simulink model "Noh_Nofusion"  (R2020b)
settings: Solver=FixedStepAuto  StartTime=0.0  StopTime=Inf  FixedStep=0.01  RelTol=1e-3
PostLoadFcn:
  | if any(exist('dsrtsu_mdlpostloadfcn', 'file') ~= 0), dsrtsu_mdlpostloadfcn('Execute', bdroot); end
InitFcn:
  | , if any(exist('rtifpga_mdlclblib', 'file') ~= 0), rtifpga_mdlclblib('Init', bdroot); end,
  | , if any(exist('dsmpb_private', 'file') ~= 0), dsmpb_private('dsmpb_mdlclblib', 'Init', bdroot); end,
undefined symbols (not defined in the file): ACC_TimeGap_DecSetSwt, ACC_TimeGap_IncSetSwt, AccelPedalPosn, AccelPedalPosnVldty, AccelPedlPosnDiagc, AccPedalOverride, ACU_ShiftInProgress, ADAS_Posn_CurLane, AESSwtReq, ALC_SwtReq, BrkPedalSts, CC_ACC_CANCEL_OFFSwt, CC_ACC_CRUISE_OFFSwt, CC_ACC_DecSetSpd_SetSwt, CC_ACC_IncSetSpd_ResuSwt, CC_ACCSwtErr, CharSpd_ms, CSA_NODE, CURRENT_GEAR, CurrentGearValid, DiscIntNeverNeededParam, DrvDoorSts, DrvSBR, DrvTrqReqOvld, ECMACCInterface, ECMRespACC, ELKSwtReq, EngLimpHomeSts, EngSpd, EngState, EngState_PHEV, EngTrqMaxActSpd, EngTrqMinAct, EPS_DrvInpTrqVal_HighReslolution, EPS_FailSts, EPS_LKATorqOvrlDlvd, EPS_LKATorqOvrlDlvdVld, EPS_LKATrqOvlDlvdSts, EPS_SteerMod, EPS_TrqSnsrSts, EQ4_APPINFO, EQ4_LA_ELEM, EQ4_LA_HDR, EQ4_LAP_ELEM, EQ4_LAP_HDR, EQ4_LH_ELEM, EQ4_LH_HDR, EQ4_LRE_ELEM, EQ4_LRE_HDR, ESS_PedSwtReq, ESS_VehSwtReq, FFogLmpSts_F_Pbox, FLWheelDriveDirection, FLWheelSpd, FrntWiprSwtSts, FrntWshrSwtSts, FRWheelDriveDirection, FRWheelSpd, HazardLmpSwtSts, HCU_AccelPedalPosn_Diag ... (+153)
libraries: simulink x132, dsmpblib x27
(part 4 of 14)

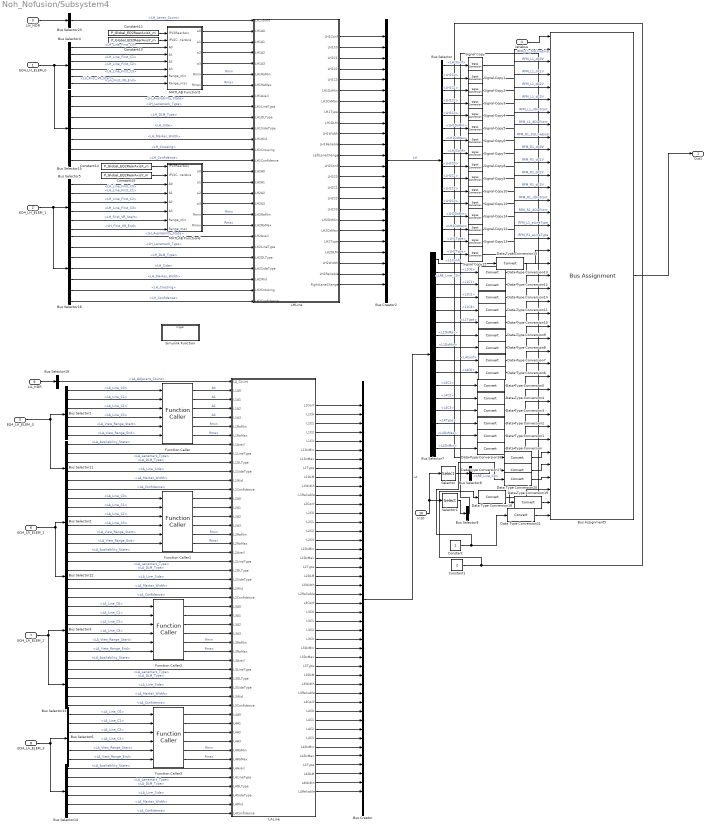
== system Noh_Nofusion/Subsystem4 ==
  EQ4_LH_ELEM_0 : Inport
  EQ4_LH_ELEM_1 : Inport  Port=2
  LH_HDR : Inport  Port=3
  lanebus : Inport  Port=4
  EQ4_LA_ELEM_0 : Inport  Port=5
  EQ4_LA_ELEM_1 : Inport  Port=6
  EQ4_LA_ELEM_2 : Inport  Port=7
  EQ4_LA_ELEM_3 : Inport  Port=8
  LA_HDR : Inport  Port=9
  In10 : Inport  Port=10
  Bus Assignment5 : BusAssignment  AssignedSignals=RFM_LINE_L1.bIsLineExist,RFM_LINE_L1.dC0V,RFM_LINE_L1.dC1V,RFM_LINE_L1.dC2V,RFM_LINE_L1.dC3V,RFM_LINE_L1.dDisStart,RFM_LINE_L1.dDisFront,RFM_LINE_R1.bIsLineExist,RFM_LINE_R1.dC0V,RFM_LINE_R1.dC1V,RFM_LINE_R1.dC2V,RFM_LINE_R1.dC3V,RFM_LINE_R1.dDisStart,RFM_LINE_R1.dDisFront,RFM_LINE_L1.eLineType,RFM_LINE_R1.eLineType,RFM_LINE_L2.bIsLineExist,RFM_LINE_L2.dC0V,RFM_LINE_L2.dC1V,RFM_LINE_L2.dC2V,RFM_LINE_L2.dC3V,RFM_LINE_L2.eLineType,RFM_LINE_L2.dDisFront,RFM_LINE_L2.dDisStart,RFM_LINE_R2.bIsLineExist,RFM_LINE_R2.dC0V,RFM_LINE_R2.dC1V,RFM_LINE_R2.dC2V,RFM_LINE_R2.dC3V,RFM_LINE_R2.eLineType,RFM_LINE_R2.dDisStart,RFM_LINE_R2.dDisFront,RFM_LINE_LB.bIsLineExist,RFM_LINE_LB.dC0V,RFM_LINE_LB.eLineType,RFM_LINE_RB.bIsLineExist,RFM_LINE_RB.dC0V,RFM_LINE_RB.eLineType
  Bus Creator : BusCreator  Inputs=44
  Bus Creator2 : BusCreator  Inputs=24
  Bus Selector : BusSelector  OutputSignals=LH1Conf,LH1C0,LH1C1,LH1C2,LH1C3,LH1DxMin,LH1DxMax,LH2Conf,LH2C0,LH2C1,LH2C2,LH2C3,LH2DxMin,LH2DxMax,LH1Type,LH2Type
  Bus Selector{1..3,6} (4 alike) : BusSelector  OutputSignals=LA_Line_C0,LA_Line_C1,LA_Line_C2,LA_Line_C3,LA_View_Range_Start,LA_View_Range_End
  Bus Selector{11..14} (4 alike) : BusSelector  OutputSignals=LA_Availability_State,LA_Lanemark_Type,LA_DLM_Type,LA_Line_Side,LA_Marker_Width,LA_Confidence
  Bus Selector15 : BusSelector  OutputSignals=LH_Availability_State,LH_Lanemark_Type,LH_DLM_Type,LH_Side,LH_Marker_Width,LH_Crossing,LH_Confidence
  Bus Selector16 : BusSelector  OutputSignals=LH_Availability_State,LH_Lanemark_Type,LH_DLM_Type,LH_Side,LH_Marker_Width,LH_Crossing,LH_Confidence
  Bus Selector19 : BusSelector  OutputSignals=LA_Adjacent_Count
  Bus Selector23 : BusSelector  OutputSignals=LH_Lanes_Count
  Bus Selector4 : BusSelector  OutputSignals=LH_Line_First_C0,LH_Line_First_C1,LH_Line_First_C2,LH_Line_First_C3,LH_First_VR_Start,LH_First_VR_End
  Bus Selector5 : BusSelector  OutputSignals=LH_Line_First_C0,LH_Line_First_C1,LH_Line_First_C2,LH_Line_First_C3,LH_First_VR_Start,LH_First_VR_End
  Bus Selector7 : BusSelector  OutputSignals=L1Conf,L1C0,L1C1,L1C2,L1C3,L1Type,L1DxMax,L1DxMin,L4Conf,L4C0,L4C1,L4C2,L4C3,L4Type,L4DxMax,L4DxMin
  Bus Selector8 : BusSelector  OutputSignals=LRE_Availability_State,LRE_Line_C0,LRE_Type
  Bus Selector9 : BusSelector  OutputSignals=LRE_Availability_State,LRE_Line_C0,LRE_Type
  Constant : Constant
  Constant1 : Constant  Value=2
  Constant12 : Constant  Value=P_Global_EQ2RearAxisX_m
  Constant13 : Constant  Value=P_Global_EQ2RearAxisY_m
  Constant14 : Constant  Value=P_Global_EQ2RearAxisX_m
  Constant15 : Constant  Value=P_Global_EQ2RearAxisY_m
  Data Type Conversion{,1..21} (22 alike) : DataTypeConversion
  Function Caller{,1..3} (4 alike) : FunctionCaller  FunctionPrototype=[a0,a1,a2,a3,Rmin,Rmax] = fla(A0,A1,A2,A3,Range_min,Range_max)  InputArgumentSpecifications=<Enter example>  OutputArgumentSpecifications=<Enter example>
  LALine : MATLAB Function  TreatAsAtomicUnit=on
  LHLine : MATLAB Function  TreatAsAtomicUnit=on
  MATLAB Function5 : MATLAB Function  TreatAsAtomicUnit=on
  MATLAB Function6 : MATLAB Function  TreatAsAtomicUnit=on
  Selector : Selector  InputPortWidth=2  IndexOptions=Index vector (dialog)  Indices=1  OutputSizes=1
  Selector1 : Selector  InputPortWidth=2  IndexOptions=Index vector (dialog)  Indices=2  OutputSizes=1
  Signal Copy{,1..15} (16 alike) : SignalConversion  OverrideOpt=off
  Simulink Function : Subsystem  TreatAsAtomicUnit=on
  Out1 : Outport
  wires:
  Constant13/1 -> MATLAB Function5/2(IFV2CenterAxis)
  LHLine/15(LH2C1) -> Bus Creator2/15
  LHLine/5(LH1C3) -> Bus Creator2/5
  MATLAB Function6/3(a2) -> LHLine/17(LH2A2)
  LHLine/17(LH2C3) -> Bus Creator2/17
  MATLAB Function6/6(Rmax) -> LHLine/20(LH2RaMax)  "Rmax"
  Bus Selector16/2 -> LHLine/22(LH2LineType)  "<LH_Lanemark_Type>"
  EQ4_LH_ELEM_1/1 -> Bus Selector16/1, Bus Selector5/1
  MATLAB Function5/6(Rmax) -> LHLine/7(LH1RaMax)  "Rmax"
  Bus Selector16/6 -> LHLine/26(LH2Crossing)  "<LH_Crossing>"
  LHLine/23(LH2Reliable) -> Bus Creator2/23
  Bus Selector15/5 -> LHLine/12(LH1Wid)  "<LH_Marker_Width>"
  LHLine/1(LH1Conf) -> Bus Creator2/1
  Constant15/1 -> MATLAB Function6/2(IFV2CenterAxis)
  EQ4_LH_ELEM_0/1 -> Bus Selector15/1, Bus Selector4/1
  Bus Selector16/3 -> LHLine/23(LH2DLType)  "<LH_DLM_Type>"
  MATLAB Function5/2(a1) -> LHLine/3(LH1A1)
  Bus Selector16/7 -> LHLine/27(LH2Confidence)  "<LH_Confidence>"
  LHLine/12(LeftLaneChange) -> Bus Creator2/12
  LHLine/9(LH1DLM) -> Bus Creator2/9
  Bus Selector15/4 -> LHLine/11(LH1SideType)  "<LH_Side>"
  LHLine/7(LH1DxMax) -> Bus Creator2/7
  LHLine/22(LH2Width) -> Bus Creator2/22
  LH_HDR/1 -> Bus Selector23/1
  Bus Selector16/1 -> LHLine/21(LH2Avail)  "<LH_Availability_State>"
  Bus Selector15/7 -> LHLine/14(LH1Confidence)  "<LH_Confidence>"
  Bus Selector4/2 -> MATLAB Function5/4(A1)  "<LH_Line_First_C1>"
  Bus Selector4/3 -> MATLAB Function5/5(A2)  "<LH_Line_First_C2>"
  Bus Selector16/5 -> LHLine/25(LH2Wid)  "<LH_Marker_Width>"
  MATLAB Function6/5(Rmin) -> LHLine/19(LH2RaMin)  "Rmin"
  LHLine/18(LH2DxMin) -> Bus Creator2/18
  LHLine/3(LH1C1) -> Bus Creator2/3
  Bus Selector5/1 -> MATLAB Function6/3(A0)  "<LH_Line_First_C0>"
  Bus Selector5/4 -> MATLAB Function6/6(A3)  "<LH_Line_First_C3>"
  Bus Selector4/4 -> MATLAB Function5/6(A3)  "<LH_Line_First_C3>"
  Bus Selector23/1 -> LHLine/1(LH_Count)  "<LH_Lanes_Count>"
  LHLine/14(LH2C0) -> Bus Creator2/14
  Bus Selector15/1 -> LHLine/8(LH1Avail)  "<LH_Availability_State>"
  MATLAB Function6/1(a0) -> LHLine/15(LH2A0)
  LHLine/8(LH1Type) -> Bus Creator2/8
  Bus Selector5/3 -> MATLAB Function6/5(A2)  "<LH_Line_First_C2>"
  MATLAB Function5/1(a0) -> LHLine/2(LH1A0)
  Bus Selector15/2 -> LHLine/9(LH1LineType)  "<LH_Lanemark_Type>"
  Bus Selector4/6 -> MATLAB Function5/8(Range_max)  "<LH_First_VR_End>"
  Constant12/1 -> MATLAB Function5/1(IFV2RearAxis)
  LHLine/4(LH1C2) -> Bus Creator2/4
  Bus Selector4/5 -> MATLAB Function5/7(Range_min)  "<LH_First_VR_Start>"
  MATLAB Function5/5(Rmin) -> LHLine/6(LH1RaMin)  "Rmin"
  MATLAB Function5/3(a2) -> LHLine/4(LH1A2)
  LHLine/11(LH1Reliable) -> Bus Creator2/11
  LHLine/20(LH2Type) -> Bus Creator2/20
  LHLine/19(LH2DxMax) -> Bus Creator2/19
  Bus Selector15/6 -> LHLine/13(LH1Crossing)  "<LH_Crossing>"
  LHLine/13(LH2Conf) -> Bus Creator2/13
  LHLine/21(LH2DLM) -> Bus Creator2/21
  LHLine/2(LH1C0) -> Bus Creator2/2
  Bus Selector16/4 -> LHLine/24(LH2SideType)  "<LH_Side>"
  Bus Selector15/3 -> LHLine/10(LH1DLType)  "<LH_DLM_Type>"
  LHLine/24(RightLaneChange) -> Bus Creator2/24
  Constant14/1 -> MATLAB Function6/1(IFV2RearAxis)
  Bus Selector4/1 -> MATLAB Function5/3(A0)  "<LH_Line_First_C0>"
  LHLine/10(LH1Width) -> Bus Creator2/10
  Bus Selector5/5 -> MATLAB Function6/7(Range_min)  "<LH_First_VR_Start>"
  MATLAB Function5/4(a3) -> LHLine/5(LH1A3)
  Bus Selector5/2 -> MATLAB Function6/4(A1)  "<LH_Line_First_C1>"
  Bus Selector5/6 -> MATLAB Function6/8(Range_max)  "<LH_First_VR_End>"
  MATLAB Function6/2(a1) -> LHLine/16(LH2A1)
  LHLine/16(LH2C2) -> Bus Creator2/16
  MATLAB Function6/4(a3) -> LHLine/18(LH2A3)
  LHLine/6(LH1DxMin) -> Bus Creator2/6
  Bus Creator2/1 -> Bus Selector/1  "LH"
  lanebus/1 -> Bus Assignment5/1
  Bus Selector/7 -> Signal Copy6/1  "<LH1DxMax>"
  Bus Selector/8 -> Signal Copy7/1  "<LH2Conf>"
  Bus Selector/6 -> Signal Copy5/1  "<LH1DxMin>"
  Bus Selector/9 -> Signal Copy8/1  "<LH2C0>"
  Bus Selector/5 -> Signal Copy4/1  "<LH1C3>"
  Bus Selector/10 -> Signal Copy9/1  "<LH2C1>"
  Bus Selector/4 -> Signal Copy3/1  "<LH1C2>"
  Bus Selector/11 -> Signal Copy10/1  "<LH2C2>"
  Bus Selector/3 -> Signal Copy2/1  "<LH1C1>"
  Bus Selector/12 -> Signal Copy11/1  "<LH2C3>"
  Bus Selector/2 -> Signal Copy1/1  "<LH1C0>"
  Bus Selector/13 -> Signal Copy14/1  "<LH2DxMin>"
  Bus Selector/1 -> Signal Copy/1  "<LH1Conf>"
  Bus Selector/14 -> Signal Copy12/1  "<LH2DxMax>"
  Bus Assignment5/1 -> Out1/1
  Bus Selector/15 -> Signal Copy13/1  "<LH1Type>"
  Bus Selector/16 -> Signal Copy15/1  "<LH2Type>"
  Signal Copy/1 -> Bus Assignment5/2  "RFM_L1_bIsLineExist"
  Signal Copy1/1 -> Bus Assignment5/3  "RFM_L1_dC0V"
  Signal Copy2/1 -> Bus Assignment5/4  "RFM_L1_dC1V"
  Signal Copy5/1 -> Bus Assignment5/7  "RFM_L1_dDisStart"
  Signal Copy3/1 -> Bus Assignment5/5  "RFM_L1_dC2V"
  Signal Copy4/1 -> Bus Assignment5/6  "RFM_L1_dC3V"
  Signal Copy8/1 -> Bus Assignment5/10  "RFM_R1_dC0V"
  Signal Copy6/1 -> Bus Assignment5/8  "RFM_L1_dDisFront"
  Signal Copy7/1 -> Bus Assignment5/9  "RFM_R1_bIsLineExist"
  Signal Copy9/1 -> Bus Assignment5/11  "RFM_R1_dC1V"
  Signal Copy11/1 -> Bus Assignment5/13  "RFM_R1_dC3V"
  Signal Copy10/1 -> Bus Assignment5/12  "RFM_R1_dC2V"
  Signal Copy12/1 -> Bus Assignment5/15  "RFM_R1_dDisFront"
  Signal Copy13/1 -> Bus Assignment5/16  "RFM_L1_eLineType"
  Signal Copy14/1 -> Bus Assignment5/14  "RFM_R1_dDisStart"
  Signal Copy15/1 -> Bus Assignment5/17  "RFM_R1_eLineType"
  Function Caller3/5 -> LALine/42(L4RaMin)  "Rmin"
  Bus Selector19/1 -> LALine/1(LA_Count)  "<LA_Adjacent_Count>"
  Bus Selector14/3 -> LALine/46(L4DLType)  "<LA_DLM_Type>"
  Bus Selector14/1 -> LALine/44(L4Avail)  "<LA_Availability_State>"
  Bus Selector13/3 -> LALine/34(L3DLType)  "<LA_DLM_Type>"
  Bus Selector14/2 -> LALine/45(L4LineType)  "<LA_Lanemark_Type>"
  Bus Selector13/5 -> LALine/36(L3Wid)  "<LA_Marker_Width>"
  Bus Selector12/5 -> LALine/24(L2Wid)  "<LA_Marker_Width>"
  Function Caller/1 -> LALine/2(L1A0)  "A0"
  Bus Selector1/5 -> Function Caller/5  "<LA_View_Range_Start>"
  Bus Selector13/1 -> LALine/32(L3Avail)  "<LA_Availability_State>"
  EQ4_LA_ELEM_3/1 -> Bus Selector14/1, Bus Selector6/1
  Function Caller2/4 -> LALine/29(L3A3)
  Function Caller3/6 -> LALine/43(L4RaMax)  "Rmax"
  Function Caller1/6 -> LALine/19(L2RaMax)  "Rmax"
  Bus Selector2/4 -> Function Caller1/4  "<LA_Line_C3>"
  Function Caller/4 -> LALine/5(L1A3)  "A3"
  Bus Selector3/6 -> Function Caller2/6  "<LA_View_Range_End>"
  Function Caller/6 -> LALine/7(L1RaMax)  "Rmax"
  Function Caller/3 -> LALine/4(L1A2)  "A2"
  Bus Selector3/3 -> Function Caller2/3  "<LA_Line_C2>"
  Bus Selector2/1 -> Function Caller1/1  "<LA_Line_C0>"
  Bus Selector3/1 -> Function Caller2/1  "<LA_Line_C0>"
  Bus Selector3/2 -> Function Caller2/2  "<LA_Line_C1>"
  Function Caller1/2 -> LALine/15(L2A1)
  Bus Selector6/6 -> Function Caller3/6  "<LA_View_Range_End>"
  Bus Selector1/3 -> Function Caller/3  "<LA_Line_C2>"
  Function Caller3/1 -> LALine/38(L4A0)
  Bus Selector6/3 -> Function Caller3/3  "<LA_Line_C2>"
  Function Caller2/3 -> LALine/28(L3A2)
  Function Caller3/4 -> LALine/41(L4A3)
  Bus Selector1/1 -> Function Caller/1  "<LA_Line_C0>"
  Bus Selector2/5 -> Function Caller1/5  "<LA_View_Range_Start>"
  Bus Selector2/6 -> Function Caller1/6  "<LA_View_Range_End>"
  Function Caller2/5 -> LALine/30(L3RaMin)  "Rmin"
  LALine/43(L4Width) -> Bus Creator/43
  LA_HDR/1 -> Bus Selector19/1
  Bus Selector6/5 -> Function Caller3/5  "<LA_View_Range_Start>"
  Bus Selector12/4 -> LALine/23(L2SideType)  "<LA_Line_Side>"
  Bus Selector14/4 -> LALine/47(L4SideType)  "<LA_Line_Side>"
  Bus Selector11/1 -> LALine/8(L1Avail)  "<LA_Availability_State>"
  LALine/11(L1Reliable) -> Bus Creator/11
  LALine/2(L1C0) -> Bus Creator/2
  EQ4_LA_ELEM_0/1 -> Bus Selector11/1, Bus Selector1/1
  LALine/15(L2C2) -> Bus Creator/15
  Function Caller2/6 -> LALine/31(L3RaMax)  "Rmax"
  EQ4_LA_ELEM_1/1 -> Bus Selector12/1, Bus Selector2/1
  LALine/6(L1DxMin) -> Bus Creator/6
  Function Caller2/1 -> LALine/26(L3A0)
  Bus Selector11/2 -> LALine/9(L1LineType)  "<LA_Lanemark_Type>"
  Function Caller1/4 -> LALine/17(L2A3)
  LALine/24(L3C0) -> Bus Creator/24
  Function Caller3/3 -> LALine/40(L4A2)
  LALine/23(L3Conf) -> Bus Creator/23
  Function Caller3/2 -> LALine/39(L4A1)
  Bus Selector12/3 -> LALine/22(L2DLType)  "<LA_DLM_Type>"
  LALine/9(L1DLM) -> Bus Creator/9
  Function Caller1/1 -> LALine/14(L2A0)
  Bus Selector14/5 -> LALine/48(L4Wid)  "<LA_Marker_Width>"
  Bus Selector2/2 -> Function Caller1/2  "<LA_Line_C1>"
  Bus Selector3/4 -> Function Caller2/4  "<LA_Line_C3>"
  LALine/21(L2Width) -> Bus Creator/21
  LALine/1(L1Conf) -> Bus Creator/1
  LALine/22(L2Reliable) -> Bus Creator/22
  Bus Selector2/3 -> Function Caller1/3  "<LA_Line_C2>"
  LALine/31(L3DLM) -> Bus Creator/31
  Bus Selector1/4 -> Function Caller/4  "<LA_Line_C3>"
  LALine/26(L3C2) -> Bus Creator/26
  Bus Selector1/6 -> Function Caller/6  "<LA_View_Range_End>"
  LALine/5(L1C3) -> Bus Creator/5
  Bus Selector12/2 -> LALine/21(L2LineType)  "<LA_Lanemark_Type>"
  LALine/3(L1C1) -> Bus Creator/3
  Bus Selector13/4 -> LALine/35(L3SideType)  "<LA_Line_Side>"
  LALine/18(L2DxMax) -> Bus Creator/18
  LALine/4(L1C2) -> Bus Creator/4
  LALine/42(L4DLM) -> Bus Creator/42
  Function Caller1/5 -> LALine/18(L2RaMin)  "Rmin"
  LALine/13(L2C0) -> Bus Creator/13
  Bus Selector12/1 -> LALine/20(L2Avail)  "<LA_Availability_State>"
  Bus Selector11/5 -> LALine/12(L1Wid)  "<LA_Marker_Width>"
  Bus Selector6/2 -> Function Caller3/2  "<LA_Line_C1>"
  LALine/12(L2Conf) -> Bus Creator/12
  LALine/36(L4C1) -> Bus Creator/36
  LALine/41(L4Type) -> Bus Creator/41
  Function Caller/5 -> LALine/6(L1RaMin)  "Rmin"
  LALine/17(L2DxMin) -> Bus Creator/17
  Function Caller/2 -> LALine/3(L1A1)  "A1"
  LALine/16(L2C3) -> Bus Creator/16
  LALine/38(L4C3) -> Bus Creator/38
  EQ4_LA_ELEM_2/1 -> Bus Selector13/1, Bus Selector3/1
  Bus Selector13/6 -> LALine/37(L3Confidence)  "<LA_Confidence>"
  LALine/19(L2Type) -> Bus Creator/19
  LALine/40(L4DxMax) -> Bus Creator/40
  Bus Selector13/2 -> LALine/33(L3LineType)  "<LA_Lanemark_Type>"
  LALine/14(L2C1) -> Bus Creator/14
  LALine/35(L4C0) -> Bus Creator/35
  LALine/20(L2DLM) -> Bus Creator/20
  LALine/34(L4Conf) -> Bus Creator/34
  LALine/33(L3Reliable) -> Bus Creator/33
  Bus Selector6/4 -> Function Caller3/4  "<LA_Line_C3>"
  LALine/44(L4Reliable) -> Bus Creator/44
  LALine/25(L3C1) -> Bus Creator/25
  LALine/30(L3Type) -> Bus Creator/30
  LALine/27(L3C3) -> Bus Creator/27
  Bus Selector6/1 -> Function Caller3/1  "<LA_Line_C0>"
  LALine/32(L3Width) -> Bus Creator/32
  Bus Selector3/5 -> Function Caller2/5  "<LA_View_Range_Start>"
  LALine/37(L4C2) -> Bus Creator/37
  Bus Selector12/6 -> LALine/25(L2Confidence)  "<LA_Confidence>"
  LALine/28(L3DxMin) -> Bus Creator/28
  Bus Selector11/6 -> LALine/13(L1Confidence)  "<LA_Confidence>"
  LALine/8(L1Type) -> Bus Creator/8
  Bus Selector14/6 -> LALine/49(L4Confidence)  "<LA_Confidence>"
  LALine/29(L3DxMax) -> Bus Creator/29
  Bus Selector1/2 -> Function Caller/2  "<LA_Line_C1>"
  Bus Selector11/4 -> LALine/11(L1SideType)  "<LA_Line_Side>"
  Function Caller2/2 -> LALine/27(L3A1)
  LALine/39(L4DxMin) -> Bus Creator/39
  Function Caller1/3 -> LALine/16(L2A2)
  LALine/10(L1Width) -> Bus Creator/10
  Bus Selector11/3 -> LALine/10(L1DLType)  "<LA_DLM_Type>"
  LALine/7(L1DxMax) -> Bus Creator/7
  Bus Creator/1 -> Bus Selector7/1  "LA"
  Bus Selector7/8 -> Data Type Conversion8/1  "<L1DxMin>"
  Bus Selector7/7 -> Data Type Conversion9/1  "<L1DxMax>"
  Bus Selector7/9 -> Data Type Conversion7/1  "<L4Conf>"
  Bus Selector7/6 -> Data Type Conversion10/1  "<L1Type>"
  Bus Selector7/10 -> Data Type Conversion6/1  "<L4C0>"
  Bus Selector7/5 -> Data Type Conversion11/1  "<L1C3>"
  Bus Selector7/11 -> Data Type Conversion5/1  "<L4C1>"
  Bus Selector7/4 -> Data Type Conversion14/1  "<L1C2>"
  Bus Selector7/12 -> Data Type Conversion4/1  "<L4C2>"
  Bus Selector7/3 -> Data Type Conversion12/1  "<L1C1>"
  Bus Selector7/13 -> Data Type Conversion3/1  "<L4C3>"
  Bus Selector7/2 -> Data Type Conversion13/1  "<L1C0>"
  Bus Selector7/14 -> Data Type Conversion2/1  "<L4Type>"
  Bus Selector7/1 -> Data Type Conversion15/1  "<L1Conf>"
  Bus Selector7/15 -> Data Type Conversion1/1  "<L4DxMax>"
  Bus Selector7/16 -> Data Type Conversion/1  "<L4DxMin>"
  Data Type Conversion/1 -> Bus Assignment5/33
  Data Type Conversion1/1 -> Bus Assignment5/32
  Data Type Conversion2/1 -> Bus Assignment5/31
  Data Type Conversion4/1 -> Bus Assignment5/29
  Data Type Conversion5/1 -> Bus Assignment5/28
  Data Type Conversion3/1 -> Bus Assignment5/30
  Data Type Conversion8/1 -> Bus Assignment5/25
  Data Type Conversion7/1 -> Bus Assignment5/26
  Data Type Conversion6/1 -> Bus Assignment5/27
  Data Type Conversion10/1 -> Bus Assignment5/23
  Data Type Conversion9/1 -> Bus Assignment5/24
  Data Type Conversion11/1 -> Bus Assignment5/22
  Data Type Conversion12/1 -> Bus Assignment5/20
  Data Type Conversion13/1 -> Bus Assignment5/19
  Data Type Conversion14/1 -> Bus Assignment5/21
  Data Type Conversion15/1 -> Bus Assignment5/18
  In10/1 -> Selector/1, Selector1/1
  Selector/1 -> Bus Selector8/1
  Bus Selector8/2 -> Data Type Conversion17/1  "<LRE_Line_C0>"
  Selector1/1 -> Bus Selector9/1
  Bus Selector9/2 -> Data Type Conversion19/1  "<LRE_Line_C0>"
  Data Type Conversion16/1 -> Bus Assignment5/34
  Data Type Conversion17/1 -> Bus Assignment5/35
  Data Type Conversion18/1 -> Bus Assignment5/37
  Data Type Conversion19/1 -> Bus Assignment5/38
  Data Type Conversion20/1 -> Bus Assignment5/36
  Data Type Conversion21/1 -> Bus Assignment5/39
  Constant/1 -> Data Type Conversion20/1, Data Type Conversion21/1
  Constant1/1 -> Data Type Conversion18/1, Data Type Conversion16/1

== system Noh_Nofusion/TOS ==
  IfStateMBus : Inport
  IfVIEBus : Inport  Port=2
  IfVCAN : Inport  Port=3  OutDataTypeStr=Bus: VCAN_BUS
  VisMsg : Inport  Port=4
  LC_Obj : Inport  Port=5
  Bus Creator1 : BusCreator  Inputs=14
  Function-Call Generator3 : simulink/Ports & Subsystems/Function-Call Generator  sample_time=0.1  numberOfIterations=1  DisallowWideOutput=off
  Rate Transition{1..3,6..9,11,15..17,19..20,22..25} (17 alike) : RateTransition  Integrity=off  Deterministic=off
  Subsystem1 : Subsystem
  IfTOSBus : Outport
  wires:
  Rate Transition1/1 -> Subsystem1/4(visMsg)
  VisMsg/1 -> Rate Transition1/1
  Subsystem1/13(TOS_UpdateCnt) -> Rate Transition25/1
  Subsystem1/12(TOS_P0_TARGET_LINE) -> Rate Transition6/1
  Subsystem1/11(TOS_AEB_JAOBJ) -> Rate Transition24/1
  Subsystem1/10(TOS_AEB_LATOBJ) -> Rate Transition23/1
  Subsystem1/9(TOS_AEB_LONOBJ) -> Rate Transition22/1
  Subsystem1/8(TOS_LCKIE) -> Rate Transition20/1
  Subsystem1/7(TOS_ELK) -> Rate Transition19/1
  Subsystem1/6(TOS_ACCP5) -> Rate Transition17/1
  Subsystem1/5(TOS_ACCP4) -> Rate Transition16/1
  Subsystem1/4(ACCP3) -> Rate Transition15/1
  Subsystem1/3(ACCP2) -> Rate Transition11/1
  Subsystem1/2(TOS_ACCP1) -> Rate Transition8/1
  Subsystem1/1(TOS_ACCP0) -> Rate Transition7/1  "TOS_ACCP0"
  Function-Call Generator3/1 -> Subsystem1/Trigger
  Rate Transition25/1 -> Bus Creator1/13  "TOS_UpdateCnt"
  Rate Transition24/1 -> Bus Creator1/11  "TOS_AEB_JAOBJ"
  Rate Transition23/1 -> Bus Creator1/10  "TOS_AEB_LATOBJ"
  Rate Transition22/1 -> Bus Creator1/9  "TOS_AEB_LONOBJ"
  LC_Obj/1 -> Bus Creator1/14  "TOS_LC"
  Rate Transition20/1 -> Bus Creator1/8  "TOS_LCKIE"
  Rate Transition19/1 -> Bus Creator1/7  "TOS_ELK"
  Rate Transition17/1 -> Bus Creator1/6  "TOS_ACCP5"
  Rate Transition16/1 -> Bus Creator1/5  "TOS_ACCP4"
  Rate Transition15/1 -> Bus Creator1/4  "TOS_ACCP3"
  Rate Transition11/1 -> Bus Creator1/3  "TOS_ACCP2"
  Rate Transition8/1 -> Bus Creator1/2  "TOS_ACCP1"
  Rate Transition6/1 -> Bus Creator1/12  "TOS_P0_TARGET_LINE"
  Rate Transition3/1 -> Subsystem1/3(IfVCAN)
  Rate Transition2/1 -> Subsystem1/2(IfVIEBus)
  Rate Transition9/1 -> Subsystem1/1(IfStateMBus)
  IfVCAN/1 -> Rate Transition3/1
  IfVIEBus/1 -> Rate Transition2/1
  IfStateMBus/1 -> Rate Transition9/1
  Rate Transition7/1 -> Bus Creator1/1  "TOS_ACCP0"
  Bus Creator1/1 -> IfTOSBus/1  "IfTOSBus"

== system Noh_Nofusion/UDP_Received ==
  function : TriggerPort  TriggerType=function-call  VariantControl=Variant
  Data Type Conversion : DataTypeConversion
  S-Function : S-Function  FunctionName=sfun_mcuEQ4api  SFunctionDeploymentMode=off  EnableBusSupport=off
  Selector : Selector  InputPortWidth=10240  IndexOptions=Index vector (dialog)  Indices=[1:1500]  OutputSizes=1
  UDP Receive (2) : dsmpblib/Data Inport  Priority=10000
      settings: SourceProductName=dSPACE Model Interface Blockset
  visMsg : Outport
  wires:
  S-Function/2 -> visMsg/1
  Data Type Conversion/1 -> S-Function/2
  Selector/1 -> S-Function/1
  UDP Receive (2)/1 -> Selector/1
  UDP Receive (2)/3 -> Data Type Conversion/1

== system Noh_Nofusion/aeb ==
  note: AEB
      | (AutoEmergencyBrake)
  IfCANBus : Inport  OutDataTypeStr=Bus: VCAN_BUS
  IfVIEBus : Inport  Port=2
  IfVSMBus : Inport  Port=3
  IfCALBus : Inport  Port=4
  IfDIAGBus : Inport  Port=5
  IfOSMBus : Inport  Port=6
  AEB : ModelReference  Commented=on  ModelNameDialog=PubIfStateAEB_MDL.slx  SimulationMode=Normal  ModelReferenceVersion=1.6
  Bus Creator : BusCreator  Inputs=3
  Bus Creator1 : BusCreator  Inputs=4
  Bus Creator10 : BusCreator  Commented=on  Inputs=1
  Bus Creator2 : BusCreator  Inputs=28
  Bus Creator3 : BusCreator  Inputs=2
  Bus Creator4 : BusCreator  Inputs=6
  Bus Creator5 : BusCreator  Inputs=2
  Bus Creator6 : BusCreator  Inputs=5
  Bus Creator7 : BusCreator  Inputs=4
  Bus Creator8 : BusCreator  Commented=on  Inputs=3
  Bus Creator9 : BusCreator  Commented=on  Inputs=4
  Bus Selector : BusSelector  OutputSignals=BCM_NODE.BCM1_MSG.DrvDoorSts,BCM_NODE.BCM1_MSG.PassengerDoorSts
  Bus Selector11 : BusSelector  OutputSignals=HUT_NODE.HUT_FD1_MSG.AEB_PedSwtReq,HUT_NODE.HUT_FD1_MSG.AEB_VehSwtReq,HUT_NODE.HUT_FD1_MSG.AEB_JASwtReq,HUT_NODE.HUT_FD1_MSG.FCW_SnvtySet
  Bus Selector12 : BusSelector  Commented=on  OutputSignals=CR_NODE.CR_FD1_MSG.FCTB_ABA_Level,CR_NODE.CR_FD1_MSG.FCTB_ABA_Req,CR_NODE.CR_FD1_MSG.FCTB_ABP_Req
  Bus Selector13 : BusSelector  Commented=on  OutputSignals=HCU_NODE.HCU_FD1_MSG.HCU_PowertrainSts,HCU_NODE.HCU_FD1_MSG.HCU_AccelPedalPosn_Diag,HCU_NODE.HCU_FD1_MSG.HCU_AccelPedalPosn_DiagValid,HCU_NODE.HCU_FD3_MSG.HCU_DrvMod
  Bus Selector14 : BusSelector  Commented=on  OutputSignals=IBOOSTER_NODE.IBOOSTER_FD2_MSG.IB_BrkPedalAppld
  Bus Selector3 : BusSelector  OutputSignals=vxvRefMs,axvRefMs2,ayvRefMs2,kapTraj,psiDtOpt
  Bus Selector4 : BusSelector  OutputSignals=ABM_NODE.ABM1_MSG.DrvSBR,ABM_NODE.ABM1_MSG.PassSBR,ABM_NODE.ABM2_MSG.VehLgtAccel,ABM_NODE.ABM2_MSG.VehLgtAccelVld
  Bus Selector5 : BusSelector  OutputSignals=ESP_NODE.ESP_FD3_MSG.FLWheelDriveDirection,ESP_NODE.ESP_FD3_MSG.FLWheelSpdVld,ESP_NODE.ESP_FD3_MSG.FLWheelSpd,ESP_NODE.ESP_FD3_MSG.FRWheelDriveDirection,ESP_NODE.ESP_FD3_MSG.FRWheelSpdVld,ESP_NODE.ESP_FD3_MSG.FRWheelSpd,ESP_NODE.ESP_FD3_MSG.RLWheelDriveDirection,ESP_NODE.ESP_FD3_MSG.RLWheelSpdVld,ESP_NODE.ESP_FD3_MSG.RRWheelSpdVld,ESP_NODE.ESP_FD3_MSG.RRWheelSpd,ESP_NODE.ESP_FD2_MSG.BTCActv,ESP_NODE.ESP_FD2_MSG.PTCActv,ESP_NODE.ESP_FD2_MSG.VDCActv,ESP_NODE.ESP_FD2_MSG.ESP_MasterCylBrkPressVld,ESP_NODE.ESP_FD2_MSG.ESP_MasterCylBrkPress,ESP_NODE.ESP_FD2_MSG.VehStandstill,ESP_NODE.ESP_FD2_MSG.ABAactv,ESP_NODE.ESP_FD2_MSG.ABAavailable,ESP_NODE.ESP_FD2_MSG.ABPActv,ESP_NODE.ESP_FD2_MSG.ABPAvailable,ESP_NODE.ESP_FD2_MSG.AEBAvailable,ESP_NODE.ESP_FD2_MSG.AEBBAActv,ESP_NODE.ESP_FD2_MSG.AEBIBActv,ESP_NODE.ESP_FD2_MSG.AWBActv,ESP_NODE.ESP_FD2_MSG.AWBAvailable,ESP_NODE.ESP_FD2_MSG.AVHSts,ESP_NODE.ESP_FD2_MSG.DrivingModDis,ESP_NODE.ESP_FD2_MSG.ESPFuncOffSts
  Bus Selector6 : BusSelector  Commented=on  OutputSignals=OSM_AEB_LONOBJ,OSM_AEB_LATOBJ,OSM_AEB_JAOBJ
  Bus Selector7 : BusSelector  OutputSignals=CSA_NODE.CSA1_MSG.LTurnLmpSwtSts,CSA_NODE.CSA1_MSG.RTurnLmpSwtSts,CSA_NODE.CSA2_MSG.SteerWheelAng,CSA_NODE.CSA2_MSG.SteerWheelAngSign,CSA_NODE.CSA2_MSG.SteerWheelSpd,CSA_NODE.CSA2_MSG.SteerWheelSpdSign
  Bus Selector8 : BusSelector  OutputSignals=DCT_NODE.DCT5_MSG.CurrentGearValid,DCT_NODE.DCT5_MSG.CURRENT_GEAR
  Bus Selector9 : BusSelector  OutputSignals=ECM_NODE.ECM_FD1_MSG.BrkPedalSts,ECM_NODE.ECM_FD2_MSG.EngState,ECM_NODE.ECM_FD2_MSG.AccelPedalPosnVldty,ECM_NODE.ECM_FD2_MSG.AccPedalOverride,ECM_NODE.ECM_FD2_MSG.AccelPedlPosnDiagc
  Subsystem : Subsystem
  IfAEBSBus : Outport
  wires:
  Bus Creator/1 -> IfAEBSBus/1  "IfAEBSBus"
  IfVIEBus/1 -> Bus Selector3/1
  Bus Selector3/1 -> Subsystem/4(vxvRefMs)  "<vxvRefMs>"
  Bus Selector3/2 -> Subsystem/5(axvRefMs2)  "<axvRefMs2>"
  Bus Selector3/3 -> Subsystem/6(ayvRefMs2)  "<ayvRefMs2>"
  Bus Selector3/4 -> Subsystem/7(kapTraj)  "<kapTraj>"
  Bus Selector3/5 -> Subsystem/8(psiDtOpt)  "<psiDtOpt>"
  Bus Selector6/1 -> ?  "<OSM_AEB_LONOBJ>"
  Bus Selector6/2 -> ?  "<OSM_AEB_LATOBJ>"
  Bus Selector6/3 -> ?  "<OSM_AEB_JAOBJ>"
  Bus Selector4/1 -> Bus Creator1/1  "<DrvSBR>"
  Bus Selector4/2 -> Bus Creator1/2  "<PassSBR>"
  Bus Selector4/3 -> Bus Creator1/3  "<VehLgtAccel>"
  Bus Selector4/4 -> Bus Creator1/4  "<VehLgtAccelVld>"
  Bus Selector5/5 -> Bus Creator2/5  "<FRWheelSpdVld>"
  Bus Selector5/4 -> Bus Creator2/4  "<FRWheelDriveDirection>"
  Bus Selector5/6 -> Bus Creator2/6  "<FRWheelSpd>"
  Bus Selector5/3 -> Bus Creator2/3  "<FLWheelSpd>"
  Bus Selector5/7 -> Bus Creator2/7  "<RLWheelDriveDirection>"
  Bus Selector5/2 -> Bus Creator2/2  "<FLWheelSpdVld>"
  Bus Selector5/8 -> Bus Creator2/8  "<RLWheelSpdVld>"
  Bus Selector5/1 -> Bus Creator2/1  "<FLWheelDriveDirection>"
  Bus Selector5/9 -> Bus Creator2/9  "<RRWheelSpdVld>"
  Bus Selector5/10 -> Bus Creator2/10  "<RRWheelSpd>"
  Bus Selector5/11 -> Bus Creator2/11  "<BTCActv>"
  Bus Selector5/12 -> Bus Creator2/12  "<PTCActv>"
  Bus Selector5/13 -> Bus Creator2/13  "<VDCActv>"
  Bus Selector5/14 -> Bus Creator2/14  "<ESP_MasterCylBrkPressVld>"
  Bus Selector5/15 -> Bus Creator2/15  "<ESP_MasterCylBrkPress>"
  Bus Selector5/16 -> Bus Creator2/16  "<VehStandstill>"
  Bus Selector5/17 -> Bus Creator2/17  "<ABAactv>"
  Bus Selector5/18 -> Bus Creator2/18  "<ABAavailable>"
  Bus Selector5/19 -> Bus Creator2/19  "<ABPActv>"
  Bus Selector5/20 -> Bus Creator2/20  "<ABPAvailable>"
  Bus Selector5/21 -> Bus Creator2/21  "<AEBAvailable>"
  Bus Selector5/22 -> Bus Creator2/22  "<AEBBAActv>"
  Bus Selector5/23 -> Bus Creator2/23  "<AEBIBActv>"
  Bus Selector5/24 -> Bus Creator2/24  "<AWBActv>"
  Bus Selector5/25 -> Bus Creator2/25  "<AWBAvailable>"
  Bus Selector5/26 -> Bus Creator2/26  "<AVHSts>"
  Bus Selector5/27 -> Bus Creator2/27  "<DrivingModDis>"
  Bus Selector5/28 -> Bus Creator2/28  "<ESPFuncOffSts>"
  Bus Selector/1 -> Bus Creator3/1  "<DrvDoorSts>"
  Bus Selector/2 -> Bus Creator3/2  "<PassengerDoorSts>"
  IfCANBus/1 -> Bus Selector4/1, Bus Selector5/1, Bus Selector14/1, Bus Selector13/1, Bus Selector12/1, Bus Selector11/1, Bus Selector9/1, Bus Selector8/1, Bus Selector7/1, Bus Selector/1
  Bus Selector7/1 -> Bus Creator4/1  "<LTurnLmpSwtSts>"
  Bus Selector7/2 -> Bus Creator4/2  "<RTurnLmpSwtSts>"
  Bus Selector7/3 -> Bus Creator4/3  "<SteerWheelAng>"
  Bus Selector7/4 -> Bus Creator4/4  "<SteerWheelAngSign>"
  Bus Selector7/5 -> Bus Creator4/5  "<SteerWheelSpd>"
  Bus Selector7/6 -> Bus Creator4/6  "<SteerWheelSpdSign>"
  Bus Selector8/1 -> Bus Creator5/1  "<CurrentGearValid>"
  Bus Selector8/2 -> Bus Creator5/2  "<CURRENT_GEAR>"
  Bus Selector9/1 -> Bus Creator6/1  "<BrkPedalSts>"
  Bus Selector9/2 -> Bus Creator6/2  "<EngState>"
  Bus Selector9/3 -> Bus Creator6/3  "<AccelPedalPosnVldty>"
  Bus Selector9/4 -> Bus Creator6/4  "<AccPedalOverride>"
  Bus Selector9/5 -> Bus Creator6/5  "<AccelPedlPosnDiagc>"
  Bus Selector11/1 -> Bus Creator7/1  "<AEB_PedSwtReq>"
  Bus Selector11/2 -> Bus Creator7/2  "<AEB_VehSwtReq>"
  Bus Selector11/3 -> Bus Creator7/3  "<AEB_JASwtReq>"
  Bus Selector11/4 -> Bus Creator7/4  "<FCW_SnvtySet>"
  Bus Selector12/1 -> Bus Creator8/1  "<FCTB_ABA_Level>"
  Bus Selector12/2 -> Bus Creator8/2  "<FCTB_ABA_Req>"
  Bus Selector12/3 -> Bus Creator8/3  "<FCTB_ABP_Req>"
  Bus Creator8/1 -> Subsystem/16(AEB_VCAN_CR)
  Bus Selector13/1 -> Bus Creator9/1  "<HCU_PowertrainSts>"
  Bus Selector13/2 -> Bus Creator9/2  "<HCU_AccelPedalPosn_Diag>"
  Bus Selector13/3 -> Bus Creator9/3  "<HCU_AccelPedalPosn_DiagValid>"
  Bus Selector13/4 -> Bus Creator9/4  "<HCU_DrvMod>"
  Bus Creator9/1 -> Subsystem/17(AEB_VCAN_HCU)
  Bus Creator10/1 -> Subsystem/18(AEB_IB_BrkPedalAppld)
  Bus Selector14/1 -> Bus Creator10/1  "<IB_BrkPedalAppld>"
  Subsystem/1(AEB_BRK_INFO) -> Bus Creator/1  "AEB_BRK_INFO"
  Subsystem/2(AEB_DVR_INFO) -> Bus Creator/2  "AEB_DVR_INFO"
  Subsystem/3(AEB_IPHUT_INFO) -> Bus Creator/3  "AEB_IPHUT_INFO"

== system Noh_Nofusion/CR_RSDS_Input/CR_L_Bus ==
  Enable : EnablePort
  Bus Creator : BusCreator  Inputs=9
  Bus Selector : BusSelector  OutputSignals=CR_L_Obj1.CR_L_ObjID_1 Value,CR_L_Obj2.CR_L_ObjID_2 Value,CR_L_Obj3.CR_L_ObjID_3 Value,CR_L_Obj4.CR_L_ObjID_4 Value,CR_L_Obj5.CR_L_ObjID_5 Value,CR_L_Obj6.CR_L_ObjID_6 Value
  Bus Selector1 : BusSelector  OutputSignals=CR_L_Obj1.CR_L_ObjDistX_1 Value,CR_L_Obj2.CR_L_ObjDistX_2 Value,CR_L_Obj3.CR_L_ObjDistX_3 Value,CR_L_Obj4.CR_L_ObjDistX_4 Value,CR_L_Obj5.CR_L_ObjDistX_5 Value,CR_L_Obj6.CR_L_ObjDistX_6 Value
  Bus Selector2 : BusSelector  OutputSignals=CR_L_Obj1.CR_L_ObjDistY_1 Value,CR_L_Obj2.CR_L_ObjDistY_2 Value,CR_L_Obj3.CR_L_ObjDistY_3 Value,CR_L_Obj4.CR_L_ObjDistY_4 Value,CR_L_Obj5.CR_L_ObjDistY_5 Value,CR_L_Obj6.CR_L_ObjDistY_6 Value
  Bus Selector3 : BusSelector  OutputSignals=CR_L_Obj1.CR_L_ObjRelVelX_1 Value,CR_L_Obj2.CR_L_ObjRelVelX_2 Value,CR_L_Obj3.CR_L_ObjRelVelX_3 Value,CR_L_Obj4.CR_L_ObjRelVelX_4 Value,CR_L_Obj5.CR_L_ObjRelVelX_5 Value,CR_L_Obj6.CR_L_ObjRelVelX_6 Value
  Bus Selector4 : BusSelector  OutputSignals=CR_L_Obj1.CR_L_ObjRelVelY_1 Value,CR_L_Obj2.CR_L_ObjRelVelY_2 Value,CR_L_Obj3.CR_L_ObjRelVelY_3 Value,CR_L_Obj4.CR_L_ObjRelVelY_4 Value,CR_L_Obj5.CR_L_ObjRelVelY_5 Value,CR_L_Obj6.CR_L_ObjRelVelY_6 Value
  Bus Selector5 : BusSelector  OutputSignals=CR_L_Obj1.CR_L_ObjRelAccelX_1 Value,CR_L_Obj2.CR_L_ObjRelAccelX_2 Value,CR_L_Obj3.CR_L_ObjRelAccelX_3 Value,CR_L_Obj4.CR_L_ObjRelAccelX_4 Value,CR_L_Obj5.CR_L_ObjRelAccelX_5 Value,CR_L_Obj6.CR_L_ObjRelAccelX_6 Value
  CL : MATLAB Function  TreatAsAtomicUnit=on
  CR_Left_Obj : dsmpblib/Data Inport  Priority=10000
      settings: SourceProductName=dSPACE Model Interface Blockset
  Constant : Constant  Value=uint8(1)  OutDataTypeStr=uint8
  Data Type Conversion{,1..5} (6 alike) : DataTypeConversion
  Mux{,1..5} (6 alike) : Mux  Inputs=6
  Terminator : Terminator
  Unit Delay : UnitDelay  SampleTime=-1  HasFrameUpgradeWarning=on
  Unit Delay1 : UnitDelay  SampleTime=-1  HasFrameUpgradeWarning=on
  CR_L_Obj : Outport
  wires:
  CR_Left_Obj/1 -> [CR_L_Obj]
  Bus Selector/1 -> Mux/1  "<CR_L_ObjID_1 Value>"
  Bus Selector/2 -> Mux/2  "<CR_L_ObjID_2 Value>"
  Bus Selector/3 -> Mux/3  "<CR_L_ObjID_3 Value>"
  Bus Selector/4 -> Mux/4  "<CR_L_ObjID_4 Value>"
  Bus Selector/5 -> Mux/5  "<CR_L_ObjID_5 Value>"
  Bus Selector/6 -> Mux/6  "<CR_L_ObjID_6 Value>"
  [CR_L_Obj] -> Bus Selector/1
  [CR_L_Obj] -> Bus Selector1/1
  Bus Selector1/6 -> Mux1/6  "<CR_L_ObjDistX_6 Value>"
  Bus Selector1/5 -> Mux1/5  "<CR_L_ObjDistX_5 Value>"
  Bus Selector1/4 -> Mux1/4  "<CR_L_ObjDistX_4 Value>"
  Bus Selector1/3 -> Mux1/3  "<CR_L_ObjDistX_3 Value>"
  Bus Selector1/2 -> Mux1/2  "<CR_L_ObjDistX_2 Value>"
  Bus Selector1/1 -> Mux1/1  "<CR_L_ObjDistX_1 Value>"
  Bus Selector2/1 -> Mux2/1  "<CR_L_ObjDistY_1 Value>"
  Bus Selector2/2 -> Mux2/2  "<CR_L_ObjDistY_2 Value>"
  Bus Selector2/3 -> Mux2/3  "<CR_L_ObjDistY_3 Value>"
  Bus Selector2/4 -> Mux2/4  "<CR_L_ObjDistY_4 Value>"
  Bus Selector2/5 -> Mux2/5  "<CR_L_ObjDistY_5 Value>"
  Bus Selector2/6 -> Mux2/6  "<CR_L_ObjDistY_6 Value>"
  [CR_L_Obj] -> Bus Selector2/1
  [CR_L_Obj] -> Bus Selector3/1
  Bus Selector3/6 -> Mux3/6  "<CR_L_ObjRelVelX_6 Value>"
  Bus Selector3/5 -> Mux3/5  "<CR_L_ObjRelVelX_5 Value>"
  Bus Selector3/4 -> Mux3/4  "<CR_L_ObjRelVelX_4 Value>"
  Bus Selector3/3 -> Mux3/3  "<CR_L_ObjRelVelX_3 Value>"
  Bus Selector3/2 -> Mux3/2  "<CR_L_ObjRelVelX_2 Value>"
  Bus Selector3/1 -> Mux3/1  "<CR_L_ObjRelVelX_1 Value>"
  Bus Selector4/1 -> Mux4/1  "<CR_L_ObjRelVelY_1 Value>"
  Bus Selector4/2 -> Mux4/2  "<CR_L_ObjRelVelY_2 Value>"
  Bus Selector4/3 -> Mux4/3  "<CR_L_ObjRelVelY_3 Value>"
  Bus Selector4/4 -> Mux4/4  "<CR_L_ObjRelVelY_4 Value>"
  Bus Selector4/5 -> Mux4/5  "<CR_L_ObjRelVelY_5 Value>"
  Bus Selector4/6 -> Mux4/6  "<CR_L_ObjRelVelY_6 Value>"
  [CR_L_Obj] -> Bus Selector4/1
  [CR_L_Obj] -> Bus Selector5/1
  Bus Selector5/6 -> Mux5/6  "<CR_L_ObjRelAccelX_6 Value>"
  Bus Selector5/5 -> Mux5/5  "<CR_L_ObjRelAccelX_5 Value>"
  Bus Selector5/4 -> Mux5/4  "<CR_L_ObjRelAccelX_4 Value>"
  Bus Selector5/3 -> Mux5/3  "<CR_L_ObjRelAccelX_3 Value>"
  Bus Selector5/2 -> Mux5/2  "<CR_L_ObjRelAccelX_2 Value>"
  Bus Selector5/1 -> Mux5/1  "<CR_L_ObjRelAccelX_1 Value>"
  Mux/1 -> Data Type Conversion/1
  Constant/1 -> CL/1(RadarID)
  Mux1/1 -> Data Type Conversion1/1
  Mux2/1 -> Data Type Conversion2/1
  Mux3/1 -> Data Type Conversion3/1
  Mux4/1 -> Data Type Conversion4/1
  Mux5/1 -> Data Type Conversion5/1
  CL/10(ObjAge) -> Bus Creator/9, Unit Delay/1
  Unit Delay/1 -> CL/9(ObjAgeK1)
  Data Type Conversion/1 -> CL/2(ID)
  Data Type Conversion1/1 -> CL/3(Dx)
  Data Type Conversion2/1 -> CL/4(Dy)
  Data Type Conversion3/1 -> CL/5(Vx)
  Data Type Conversion4/1 -> CL/6(Vy)
  Data Type Conversion5/1 -> CL/7(Ax)
  CL/9(ObjID) -> Unit Delay1/1, Bus Creator/8
  Unit Delay1/1 -> CL/8(ObjIDK1)
  CL/1(P) -> Terminator/1
  CL/2(ObjDx) -> Bus Creator/1
  CL/3(ObjDy) -> Bus Creator/2
  CL/4(ObjVx) -> Bus Creator/3
  CL/5(ObjVy) -> Bus Creator/4
  CL/6(ObjAx) -> Bus Creator/5
  CL/7(ObjMoveSts) -> Bus Creator/6
  CL/8(ObjFusType) -> Bus Creator/7
  Bus Creator/1 -> CR_L_Obj/1

== system Noh_Nofusion/CR_RSDS_Input/CR_R_Bus ==
  Enable : EnablePort
  Bus Creator : BusCreator  Inputs=9
  Bus Selector : BusSelector  OutputSignals=CR_R_Obj1.CR_R_ObjID_1 Value,CR_R_Obj2.CR_R_ObjID_2 Value,CR_R_Obj3.CR_R_ObjID_3 Value,CR_R_Obj4.CR_R_ObjID_4 Value,CR_R_Obj5.CR_R_ObjID_5 Value,CR_R_Obj6.CR_R_ObjID_6 Value
  Bus Selector1 : BusSelector  OutputSignals=CR_R_Obj1.CR_R_ObjDistX_1 Value,CR_R_Obj2.CR_R_ObjDistX_2 Value,CR_R_Obj3.CR_R_ObjDistX_3 Value,CR_R_Obj4.CR_R_ObjDistX_4 Value,CR_R_Obj5.CR_R_ObjDistX_5 Value,CR_R_Obj6.CR_R_ObjDistX_6 Value
  Bus Selector2 : BusSelector  OutputSignals=CR_R_Obj1.CR_R_ObjDistY_1 Value,CR_R_Obj2.CR_R_ObjDistY_2 Value,CR_R_Obj3.CR_R_ObjDistY_3 Value,CR_R_Obj4.CR_R_ObjDistY_4 Value,CR_R_Obj5.CR_R_ObjDistY_5 Value,CR_R_Obj6.CR_R_ObjDistY_6 Value
  Bus Selector3 : BusSelector  OutputSignals=CR_R_Obj1.CR_R_ObjRelVelX_1 Value,CR_R_Obj2.CR_R_ObjRelVelX_2 Value,CR_R_Obj3.CR_R_ObjRelVelX_3 Value,CR_R_Obj4.CR_R_ObjRelVelX_4 Value,CR_R_Obj5.CR_R_ObjRelVelX_5 Value,CR_R_Obj6.CR_R_ObjRelVelX_6 Value
  Bus Selector4 : BusSelector  OutputSignals=CR_R_Obj1.CR_R_ObjRelVelY_1 Value,CR_R_Obj2.CR_R_ObjRelVelY_2 Value,CR_R_Obj3.CR_R_ObjRelVelY_3 Value,CR_R_Obj4.CR_R_ObjRelVelY_4 Value,CR_R_Obj5.CR_R_ObjRelVelY_5 Value,CR_R_Obj6.CR_R_ObjRelVelY_6 Value
  Bus Selector5 : BusSelector  OutputSignals=CR_R_Obj1.CR_R_ObjRelAccelX_1 Value,CR_R_Obj2.CR_R_ObjRelAccelX_2 Value,CR_R_Obj3.CR_R_ObjRelAccelX_3 Value,CR_R_Obj4.CR_R_ObjRelAccelX_4 Value,CR_R_Obj5.CR_R_ObjRelAccelX_5 Value,CR_R_Obj6.CR_R_ObjRelAccelX_6 Value
  CR : MATLAB Function  TreatAsAtomicUnit=on
  CR_Right_Obj : dsmpblib/Data Inport  Priority=10000
      settings: SourceProductName=dSPACE Model Interface Blockset
  Constant : Constant  Value=uint8(2)  OutDataTypeStr=uint8
  Data Type Conversion{,1..5} (6 alike) : DataTypeConversion
  Mux{,1..5} (6 alike) : Mux  Inputs=6
  Terminator : Terminator
  Unit Delay : UnitDelay  SampleTime=-1  HasFrameUpgradeWarning=on
  Unit Delay1 : UnitDelay  SampleTime=-1  HasFrameUpgradeWarning=on
  CR_R_Obj : Outport
  wires:
  CR_Right_Obj/1 -> [CR_R_Obj]
  Data Type Conversion5/1 -> CR/7(Ax)
  Data Type Conversion4/1 -> CR/6(Vy)
  Data Type Conversion/1 -> CR/2(ID)
  Bus Creator/1 -> CR_R_Obj/1
  Mux3/1 -> Data Type Conversion3/1
  Mux4/1 -> Data Type Conversion4/1
  CR/10(ObjAge) -> Bus Creator/9, Unit Delay/1
  Mux2/1 -> Data Type Conversion2/1
  Constant/1 -> CR/1(RadarID)
  CR/9(ObjID) -> Unit Delay1/1, Bus Creator/8
  CR/6(ObjAx) -> Bus Creator/5
  CR/8(ObjFusType) -> Bus Creator/7
  CR/7(ObjMoveSts) -> Bus Creator/6
  Bus Selector5/4 -> Mux5/4  "<CR_R_ObjRelAccelX_4 Value>"
  Mux1/1 -> Data Type Conversion1/1
  Mux/1 -> Data Type Conversion/1
  Bus Selector/3 -> Mux/3  "<CR_R_ObjID_3 Value>"
  Bus Selector1/1 -> Mux1/1  "<CR_R_ObjDistX_1 Value>"
  Bus Selector5/1 -> Mux5/1  "<CR_R_ObjRelAccelX_1 Value>"
  Data Type Conversion2/1 -> CR/4(Dy)
  [CR_R_Obj] -> Bus Selector2/1
  Bus Selector/1 -> Mux/1  "<CR_R_ObjID_1 Value>"
  Bus Selector4/5 -> Mux4/5  "<CR_R_ObjRelVelY_5 Value>"
  CR/4(ObjVx) -> Bus Creator/3
  Bus Selector4/4 -> Mux4/4  "<CR_R_ObjRelVelY_4 Value>"
  Bus Selector5/5 -> Mux5/5  "<CR_R_ObjRelAccelX_5 Value>"
  CR/1(P) -> Terminator/1
  [CR_R_Obj] -> Bus Selector5/1
  Unit Delay/1 -> CR/9(ObjAgeK1)
  [CR_R_Obj] -> Bus Selector4/1
  Bus Selector3/4 -> Mux3/4  "<CR_R_ObjRelVelX_4 Value>"
  Bus Selector3/6 -> Mux3/6  "<CR_R_ObjRelVelX_6 Value>"
  Bus Selector3/1 -> Mux3/1  "<CR_R_ObjRelVelX_1 Value>"
  Bus Selector5/2 -> Mux5/2  "<CR_R_ObjRelAccelX_2 Value>"
  CR/3(ObjDy) -> Bus Creator/2
  Bus Selector3/5 -> Mux3/5  "<CR_R_ObjRelVelX_5 Value>"
  Bus Selector2/6 -> Mux2/6  "<CR_R_ObjDistY_6 Value>"
  Bus Selector4/1 -> Mux4/1  "<CR_R_ObjRelVelY_1 Value>"
  Mux5/1 -> Data Type Conversion5/1
  [CR_R_Obj] -> Bus Selector3/1
  Unit Delay1/1 -> CR/8(ObjIDK1)
  Bus Selector5/3 -> Mux5/3  "<CR_R_ObjRelAccelX_3 Value>"
  Bus Selector4/2 -> Mux4/2  "<CR_R_ObjRelVelY_2 Value>"
  Bus Selector3/2 -> Mux3/2  "<CR_R_ObjRelVelX_2 Value>"
  Bus Selector3/3 -> Mux3/3  "<CR_R_ObjRelVelX_3 Value>"
  Bus Selector4/3 -> Mux4/3  "<CR_R_ObjRelVelY_3 Value>"
  Bus Selector2/2 -> Mux2/2  "<CR_R_ObjDistY_2 Value>"
  Bus Selector1/3 -> Mux1/3  "<CR_R_ObjDistX_3 Value>"
  Bus Selector1/6 -> Mux1/6  "<CR_R_ObjDistX_6 Value>"
  CR/5(ObjVy) -> Bus Creator/4
  Bus Selector1/2 -> Mux1/2  "<CR_R_ObjDistX_2 Value>"
  [CR_R_Obj] -> Bus Selector/1
  Bus Selector2/4 -> Mux2/4  "<CR_R_ObjDistY_4 Value>"
  Bus Selector4/6 -> Mux4/6  "<CR_R_ObjRelVelY_6 Value>"
  [CR_R_Obj] -> Bus Selector1/1
  CR/2(ObjDx) -> Bus Creator/1
  Bus Selector2/5 -> Mux2/5  "<CR_R_ObjDistY_5 Value>"
  Bus Selector1/5 -> Mux1/5  "<CR_R_ObjDistX_5 Value>"
  Bus Selector/6 -> Mux/6  "<CR_R_ObjID_6 Value>"
  Bus Selector2/1 -> Mux2/1  "<CR_R_ObjDistY_1 Value>"
  Bus Selector5/6 -> Mux5/6  "<CR_R_ObjRelAccelX_6 Value>"
  Data Type Conversion1/1 -> CR/3(Dx)
  Bus Selector/5 -> Mux/5  "<CR_R_ObjID_5 Value>"
  Bus Selector/2 -> Mux/2  "<CR_R_ObjID_2 Value>"
  Data Type Conversion3/1 -> CR/5(Vx)
  Bus Selector2/3 -> Mux2/3  "<CR_R_ObjDistY_3 Value>"
  Bus Selector1/4 -> Mux1/4  "<CR_R_ObjDistX_4 Value>"
  Bus Selector/4 -> Mux/4  "<CR_R_ObjID_4 Value>"

== system Noh_Nofusion/CR_RSDS_Input/RSDS_L_Bus ==
  Enable : EnablePort
  Bus Creator : BusCreator  Inputs=9
  Bus Selector : BusSelector  OutputSignals=RSDS_L_Obj1.RSDS_L_ObjID_1 Value,RSDS_L_Obj2.RSDS_L_ObjID_2 Value,RSDS_L_Obj3.RSDS_L_ObjID_3 Value,RSDS_L_Obj4.RSDS_L_ObjID_4 Value,RSDS_L_Obj5.RSDS_L_ObjID_5 Value,RSDS_L_Obj6.RSDS_L_ObjID_6 Value
  Bus Selector1 : BusSelector  OutputSignals=RSDS_L_Obj1.RSDS_L_ObjDistX_1 Value,RSDS_L_Obj2.RSDS_L_ObjDistX_2 Value,RSDS_L_Obj3.RSDS_L_ObjDistX_3 Value,RSDS_L_Obj4.RSDS_L_ObjDistX_4 Value,RSDS_L_Obj5.RSDS_L_ObjDistX_5 Value,RSDS_L_Obj6.RSDS_L_ObjDistX_6 Value
  Bus Selector2 : BusSelector  OutputSignals=RSDS_L_Obj1.RSDS_L_ObjDistY_1 Value,RSDS_L_Obj2.RSDS_L_ObjDistY_2 Value,RSDS_L_Obj3.RSDS_L_ObjDistY_3 Value,RSDS_L_Obj4.RSDS_L_ObjDistY_4 Value,RSDS_L_Obj5.RSDS_L_ObjDistY_5 Value,RSDS_L_Obj6.RSDS_L_ObjDistY_6 Value
  Bus Selector3 : BusSelector  OutputSignals=RSDS_L_Obj1.RSDS_L_ObjRelVelX_1 Value,RSDS_L_Obj2.RSDS_L_ObjRelVelX_2 Value,RSDS_L_Obj3.RSDS_L_ObjRelVelX_3 Value,RSDS_L_Obj4.RSDS_L_ObjRelVelX_4 Value,RSDS_L_Obj5.RSDS_L_ObjRelVelX_5 Value,RSDS_L_Obj6.RSDS_L_ObjRelVelX_6 Value
  Bus Selector4 : BusSelector  OutputSignals=RSDS_L_Obj1.RSDS_L_ObjRelVelY_1 Value,RSDS_L_Obj2.RSDS_L_ObjRelVelY_2 Value,RSDS_L_Obj3.RSDS_L_ObjRelVelY_3 Value,RSDS_L_Obj4.RSDS_L_ObjRelVelY_4 Value,RSDS_L_Obj5.RSDS_L_ObjRelVelY_5 Value,RSDS_L_Obj6.RSDS_L_ObjRelVelY_6 Value
  Bus Selector5 : BusSelector  OutputSignals=RSDS_L_Obj1.RSDS_L_ObjRelAccelX_1 Value,RSDS_L_Obj2.RSDS_L_ObjRelAccelX_2 Value,RSDS_L_Obj3.RSDS_L_ObjRelAccelX_3 Value,RSDS_L_Obj4.RSDS_L_ObjRelAccelX_4 Value,RSDS_L_Obj5.RSDS_L_ObjRelAccelX_5 Value,RSDS_L_Obj6.RSDS_L_ObjRelAccelX_6 Value
  Constant : Constant  Value=uint8(3)  OutDataTypeStr=uint8
  Data Type Conversion{,1..5} (6 alike) : DataTypeConversion
  Mux{,1..5} (6 alike) : Mux  Inputs=6
  RSDS_L : MATLAB Function  TreatAsAtomicUnit=on
  RSDS_Left_Obj : dsmpblib/Data Inport  Priority=10000
      settings: SourceProductName=dSPACE Model Interface Blockset
  Terminator : Terminator
  Unit Delay : UnitDelay  SampleTime=-1  HasFrameUpgradeWarning=on
  Unit Delay1 : UnitDelay  SampleTime=-1  HasFrameUpgradeWarning=on
  RSDS_L_Obj : Outport
  wires:
  RSDS_Left_Obj/1 -> [RSDS_L_Obj]
  Bus Selector/4 -> Mux/4  "<RSDS_L_ObjID_4 Value>"
  Bus Selector1/4 -> Mux1/4  "<RSDS_L_ObjDistX_4 Value>"
  Bus Selector2/3 -> Mux2/3  "<RSDS_L_ObjDistY_3 Value>"
  Data Type Conversion3/1 -> RSDS_L/5(Vx)
  Bus Selector/5 -> Mux/5  "<RSDS_L_ObjID_5 Value>"
  Bus Selector2/1 -> Mux2/1  "<RSDS_L_ObjDistY_1 Value>"
  Bus Selector/2 -> Mux/2  "<RSDS_L_ObjID_2 Value>"
  [RSDS_L_Obj] -> Bus Selector1/1
  Bus Selector1/5 -> Mux1/5  "<RSDS_L_ObjDistX_5 Value>"
  RSDS_L/2(ObjDx) -> Bus Creator/1
  Bus Selector2/4 -> Mux2/4  "<RSDS_L_ObjDistY_4 Value>"
  [RSDS_L_Obj] -> Bus Selector/1
  Bus Selector1/6 -> Mux1/6  "<RSDS_L_ObjDistX_6 Value>"
  Bus Selector5/6 -> Mux5/6  "<RSDS_L_ObjRelAccelX_6 Value>"
  Bus Selector1/2 -> Mux1/2  "<RSDS_L_ObjDistX_2 Value>"
  Bus Selector1/3 -> Mux1/3  "<RSDS_L_ObjDistX_3 Value>"
  Bus Selector/6 -> Mux/6  "<RSDS_L_ObjID_6 Value>"
  Bus Selector3/2 -> Mux3/2  "<RSDS_L_ObjRelVelX_2 Value>"
  Mux5/1 -> Data Type Conversion5/1
  Bus Selector4/1 -> Mux4/1  "<RSDS_L_ObjRelVelY_1 Value>"
  Bus Selector2/6 -> Mux2/6  "<RSDS_L_ObjDistY_6 Value>"
  RSDS_L/3(ObjDy) -> Bus Creator/2
  Bus Selector4/3 -> Mux4/3  "<RSDS_L_ObjRelVelY_3 Value>"
  Bus Selector3/1 -> Mux3/1  "<RSDS_L_ObjRelVelX_1 Value>"
  Bus Selector5/2 -> Mux5/2  "<RSDS_L_ObjRelAccelX_2 Value>"
  Bus Selector3/5 -> Mux3/5  "<RSDS_L_ObjRelVelX_5 Value>"
  Unit Delay1/1 -> RSDS_L/8(ObjIDK1)
  [RSDS_L_Obj] -> Bus Selector5/1
  Bus Selector5/3 -> Mux5/3  "<RSDS_L_ObjRelAccelX_3 Value>"
  Bus Selector3/4 -> Mux3/4  "<RSDS_L_ObjRelVelX_4 Value>"
  RSDS_L/1(P) -> Terminator/1
  Bus Selector5/5 -> Mux5/5  "<RSDS_L_ObjRelAccelX_5 Value>"
  Bus Selector3/6 -> Mux3/6  "<RSDS_L_ObjRelVelX_6 Value>"
  Bus Selector4/5 -> Mux4/5  "<RSDS_L_ObjRelVelY_5 Value>"
  Bus Selector4/2 -> Mux4/2  "<RSDS_L_ObjRelVelY_2 Value>"
  RSDS_L/4(ObjVx) -> Bus Creator/3
  [RSDS_L_Obj] -> Bus Selector4/1
  Data Type Conversion1/1 -> RSDS_L/3(Dx)
  Bus Selector/1 -> Mux/1  "<RSDS_L_ObjID_1 Value>"
  RSDS_L/5(ObjVy) -> Bus Creator/4
  [RSDS_L_Obj] -> Bus Selector2/1
  Data Type Conversion2/1 -> RSDS_L/4(Dy)
  Bus Selector5/1 -> Mux5/1  "<RSDS_L_ObjRelAccelX_1 Value>"
  Bus Selector1/1 -> Mux1/1  "<RSDS_L_ObjDistX_1 Value>"
  Bus Selector/3 -> Mux/3  "<RSDS_L_ObjID_3 Value>"
  Mux/1 -> Data Type Conversion/1
  [RSDS_L_Obj] -> Bus Selector3/1
  Mux1/1 -> Data Type Conversion1/1
  RSDS_L/7(ObjMoveSts) -> Bus Creator/6
  Bus Selector2/2 -> Mux2/2  "<RSDS_L_ObjDistY_2 Value>"
  RSDS_L/8(ObjFusType) -> Bus Creator/7
  Bus Selector4/4 -> Mux4/4  "<RSDS_L_ObjRelVelY_4 Value>"
  RSDS_L/6(ObjAx) -> Bus Creator/5
  Bus Selector5/4 -> Mux5/4  "<RSDS_L_ObjRelAccelX_4 Value>"
  RSDS_L/9(ObjID) -> Unit Delay1/1, Bus Creator/8
  Constant/1 -> RSDS_L/1(RadarID)
  Bus Selector3/3 -> Mux3/3  "<RSDS_L_ObjRelVelX_3 Value>"
  Bus Selector4/6 -> Mux4/6  "<RSDS_L_ObjRelVelY_6 Value>"
  Unit Delay/1 -> RSDS_L/9(ObjAgeK1)
  RSDS_L/10(ObjAge) -> Bus Creator/9, Unit Delay/1
  Mux4/1 -> Data Type Conversion4/1
  Mux2/1 -> Data Type Conversion2/1
  Bus Creator/1 -> RSDS_L_Obj/1
  Mux3/1 -> Data Type Conversion3/1
  Data Type Conversion/1 -> RSDS_L/2(ID)
  Data Type Conversion5/1 -> RSDS_L/7(Ax)
  Bus Selector2/5 -> Mux2/5  "<RSDS_L_ObjDistY_5 Value>"
  Data Type Conversion4/1 -> RSDS_L/6(Vy)
